simulink model "uncompensated_system"  (R2022a)
settings: Solver=VariableStepAuto  StartTime=0.0  StopTime=30  MaxStep=0.01  RelTol=1e-3
settings Model: Creator=charbel199  LastModifiedBy=charbel199

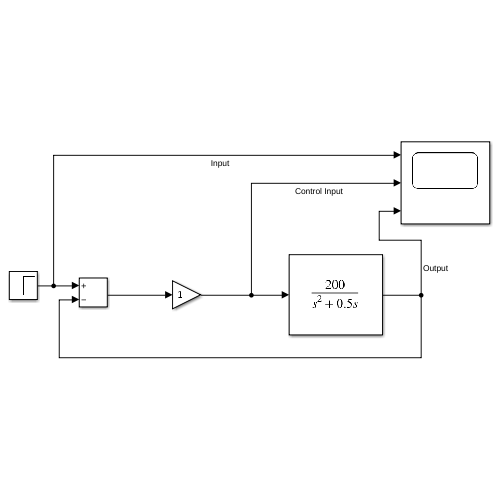
[thumbnail: Simulink's stored preview of the top-level diagram]
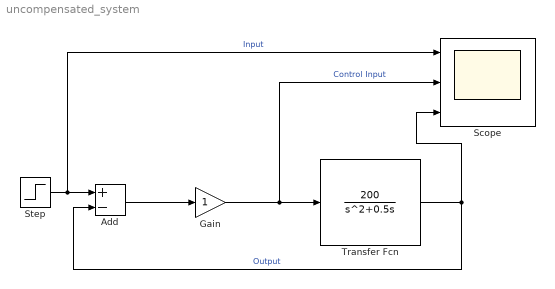
== system uncompensated_system ==
  Add : Sum  Inputs=+-
  Gain : Gain
  Scope : Scope  NumInputPorts=3
  Step : Step  After=100  SampleTime=0
  Transfer Fcn : TransferFcn  Numerator=[200]  Denominator=[1 0.5 0]
  wires:
  Step/1 -> Scope/1, Add/1  "Input"
  Add/1 -> Gain/1
  Gain/1 -> Scope/2, Transfer Fcn/1  "Control Input"
  Transfer Fcn/1 -> Add/2, Scope/3  "Output"
